simulink model "InverseDynamicsControl"  (R2021b)
settings: Solver=VariableStepAuto  StartTime=0.0  StopTime=10.0  RelTol=1e-3
undefined symbols (not defined in the file or in its folder): K_D, K_P
settings Model: Creator=ASUS  LastModifiedBy=ASUS

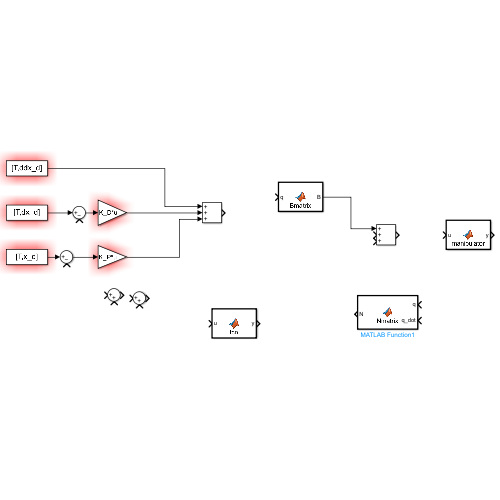
[thumbnail: Simulink's stored preview of the top-level diagram]
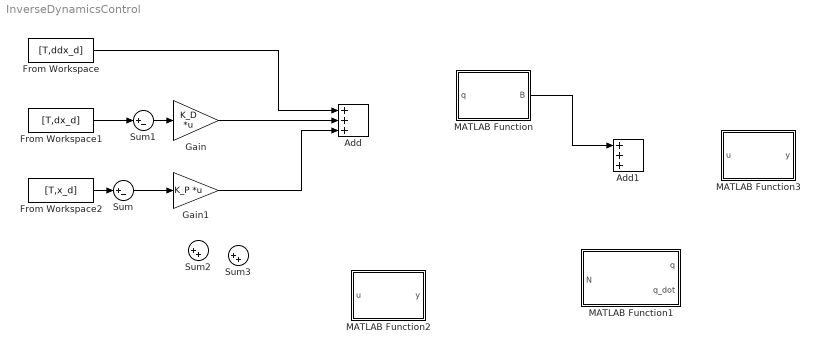
== system InverseDynamicsControl ==
  Add : Sum  Inputs=+++
  Add1 : Sum  Inputs=+++
  From Workspace : FromWorkspace  VariableName=[T,ddx_d]
  From Workspace1 : FromWorkspace  VariableName=[T,dx_d]
  From Workspace2 : FromWorkspace  VariableName=[T,x_d]
  Gain : Gain  Gain=K_D  Multiplication=Matrix(K*u)
  Gain1 : Gain  Gain=K_P  Multiplication=Matrix(K*u)
  MATLAB Function : MATLAB Function  TreatAsAtomicUnit=on
  MATLAB Function1 : MATLAB Function  TreatAsAtomicUnit=on
  MATLAB Function2 : MATLAB Function  TreatAsAtomicUnit=on
  MATLAB Function3 : MATLAB Function  TreatAsAtomicUnit=on
  Sum : Sum  Inputs=|+-
  Sum1 : Sum  Inputs=|+-
  Sum2 : Sum  Inputs=|++
  Sum3 : Sum  Inputs=|++
  wires:
  MATLAB Function/1(B) -> Add1/1
  From Workspace/1 -> Add/1
  Gain/1 -> Add/2
  Gain1/1 -> Add/3
  From Workspace2/1 -> Sum/1
  Sum/1 -> Gain1/1
  From Workspace1/1 -> Sum1/1
  Sum1/1 -> Gain/1

== matlab function InverseDynamicsControl/MATLAB Function ==
  data: q input; B output
function B  = Bmatrix(q)
B = ones(6,6);
end

== matlab function InverseDynamicsControl/MATLAB Function2 ==
  data: u input; y output
function y = fcn(u)

y = u;

== matlab function InverseDynamicsControl/MATLAB Function3 ==
  data: u input; y output
function y = manipulator(u)

y = 0;
end

== matlab function InverseDynamicsControl/MATLAB Function1 ==
  data: q input; N output; q_dot input
function N  = Nmatrix(q,q_dot)
%NMATRIX Summary of this function goes here
%   Detailed explanation goes here
N = ones(6,6);
end
